simulink model "checkDataParallel"  (Simulink 7.2)
settings: Solver=FixedStepDiscrete  StartTime=0.0  StopTime=10.0  FixedStep=0.05  RelTol=1e-3
settings Model: Creator=jrivitus  LastModifiedBy=jrivitus
settings OptimizationCC: InitFltsAndDblsToZero=on

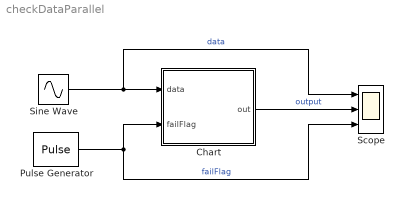
== system checkDataParallel ==
  Chart : Stateflow chart
  Pulse Generator : DiscretePulseGenerator  Period=30  SampleTime=0.05
  Scope : Scope  NumInputPorts=3
      settings: YMin=-1.1~-1.1~-0.1  YMax=1.1~1.1~1.1
  Sine Wave : Sin  SampleTime=0.05
  wires:
  Chart/1(out) -> Scope/2  "output"
  Sine Wave/1 -> Scope/1, Chart/1(data)  "data"
  Pulse Generator/1 -> Chart/2(failFlag), Scope/3  "failFlag"

== stateflow chart Chart ==
  state FailureDecision [parallel]
    settings: executionOrder=1
    state FailureOccurred
      entry:
      count = 1;
      failMode = 1;
      during:
      count++;
    state NormalOperation
      entry:
      failMode = 0;
    FailureOccurred -> FailureOccurred [order 1] : /*Reset counter*/
        | [failFlag == 1]
    FailureOccurred -> NormalOperation [order 2] : /*After 5 cycles
        |    with no failure*/
        | [count == 5]
    NormalOperation -> FailureOccurred : /*When failure occurs*/
        | [failFlag == 1]
    (default) -> NormalOperation
  state DataOutput [parallel]
    settings: executionOrder=2
    state OutputEqualsInput
      entry:
      out = data;
      during:
      out = data;
    state OutputEqualsZero
      entry:
      out = 0;
      during:
      out = 0;
    (default) -> OutputEqualsInput
    OutputEqualsInput -> OutputEqualsZero : [failMode == 1]
    OutputEqualsZero -> OutputEqualsInput : [failMode == 0]
  data: count local double; data input double; failFlag input double; out output double; failMode local double
